simulink model "building_EXAMPLE_v1"  (R2016b)
settings: Solver=ode23tb  StartTime=-building.preruntime+8760*3600  StopTime=building.runtime+8760*3600  MaxStep=600  EnableMultiTasking=on
StartFcn:
  | tic
StopFcn:
  | toc
values from neighbouring files (symbols this model uses):
  building = create_building_automatic(building, modify, import_mode, name_XML, name_EXCEL, name_PHPP, NUMBEROFZONES)    [work_EXAMPLE_v1.m]
undefined symbols (not defined in the file or in its folder): A, B, C, cp, Dd, Dreifach, FluidMix, get_building, ID, MassFlow, p, Pressure, Qdot_C, Qdot_C_energy, Qdot_H, Qdot_H_energy, Qdot_I_electricity, Qdot_I_electricity_energy, Qdot_I_light, Qdot_I_light_energy, Qdot_I_person, Qdot_I_person_energy, Qdot_S, Qdot_S_energy, Qdot_T_ground, Qdot_T_ground_energy, Qdot_T_neighbour, Qdot_T_neighbour_energy, Qdot_T_opaque, Qdot_T_opaque_energy, Qdot_T_window, Qdot_T_window_energy, Qdot_V_infiltration, Qdot_V_infiltration_energy, Qdot_V_mech, Qdot_V_mech_energy, Qdot_V_window, Qdot_V_window_energy, rho, Tc, Temperature, Tr, Ts, Wärmeschutzglas, x_CO2, x_H2O, x_VOC
libraries: carnotUIBK x1931, carnot x83, simulink_extras x22, simulink x12
(part 8 of 35)

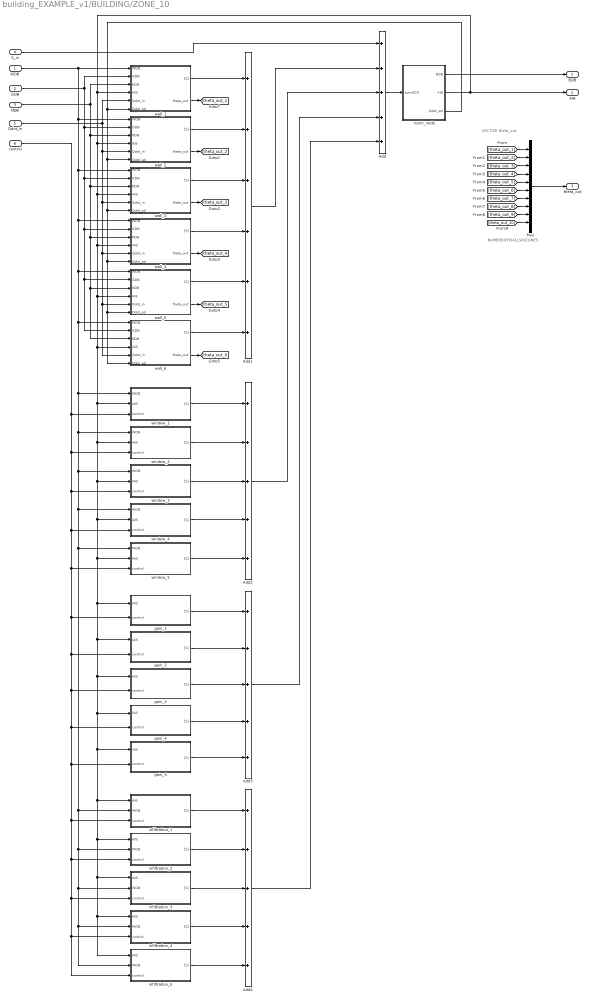
== system building_EXAMPLE_v1/BUILDING/ZONE_10 ==
  note: VECTOR theta_out
  note: NUMBEROFWALLSINZONES
  WDB : Inport
  GDB : Inport  Port=2
  NDB : Inport  Port=3
  S_in : Inport  Port=4
  Qdot_in : Inport  Port=5
  control : Inport  Port=6
  Add{,2..4} (4 alike) : Sum  Inputs=5
  Add1 : Sum  Inputs=6
  Mux : Mux  Inputs=10
  gain_1 : Subsystem  Variant=on  mask{zone=z.matrix_gains, gains=b.gains, subgain=1}
      mask init: same as building_EXAMPLE_v1/BUILDING/ZONE_1/gain_1
      mask Display:
      | fprintf('GAINS:\n')
      | fprintf('\n%s', ga.name)
  gain_2 : Subsystem  Variant=on  mask{zone=z.matrix_gains, gains=b.gains, subgain=2}
      mask init: same as building_EXAMPLE_v1/BUILDING/ZONE_1/gain_1
      mask Display:
      | fprintf('GAINS:\n')
      | fprintf('\n%s', ga.name)
  gain_3 : Subsystem  Variant=on  mask{zone=z.matrix_gains, gains=b.gains, subgain=3}
      mask init: same as building_EXAMPLE_v1/BUILDING/ZONE_1/gain_1
      mask Display:
      | fprintf('GAINS:\n')
      | fprintf('\n%s', ga.name)
  gain_4 : Subsystem  Variant=on  mask{zone=z.matrix_gains, gains=b.gains, subgain=4}
      mask init: same as building_EXAMPLE_v1/BUILDING/ZONE_1/gain_1
      mask Display:
      | fprintf('GAINS:\n')
      | fprintf('\n%s', ga.name)
  gain_5 : Subsystem  Variant=on  mask{zone=z.matrix_gains, gains=b.gains, subgain=4}
      mask init: same as building_EXAMPLE_v1/BUILDING/ZONE_1/gain_1
      mask Display:
      | fprintf('GAINS:\n')
      | fprintf('\n%s', ga.name)
  infiltration_1 : Subsystem  Variant=on  mask{zone=z.matrix_wi, window=1}
      mask init: same as building_EXAMPLE_v1/BUILDING/ZONE_1/infiltration_1
      mask Display:
      | fprintf('INFILTRATION:\n')
      | %fprintf('\n%s', const.name)
  infiltration_2 : Subsystem  Variant=on  mask{zone=z.matrix_wi, window=2}
      mask init: same as building_EXAMPLE_v1/BUILDING/ZONE_1/infiltration_1
      mask Display:
      | fprintf('INFILTRATION:\n')
      | %fprintf('\n%s', const.name)
  infiltration_3 : Subsystem  Variant=on  mask{zone=z.matrix_wi, window=3}
      mask init: same as building_EXAMPLE_v1/BUILDING/ZONE_1/infiltration_1
      mask Display:
      | fprintf('INFILTRATION:\n')
      | %fprintf('\n%s', const.name)
  infiltration_4 : Subsystem  Variant=on  mask{zone=z.matrix_wi, window=4}
      mask init: same as building_EXAMPLE_v1/BUILDING/ZONE_1/infiltration_1
      mask Display:
      | fprintf('INFILTRATION:\n')
      | %fprintf('\n%s', const.name)
  infiltration_5 : Subsystem  Variant=on  mask{zone=z.matrix_wi, window=5}
      mask init: same as building_EXAMPLE_v1/BUILDING/ZONE_1/infiltration_1
      mask Display:
      | fprintf('INFILTRATION:\n')
      | %fprintf('\n%s', const.name)
  room_node : Subsystem  Variant=on
  wall_1 : Subsystem  Variant=on  mask{zone=z.matrix_wd, construction=b.construction, wall=1}
      mask init: same as building_EXAMPLE_v1/BUILDING/ZONE_1/wall_1
      mask Display:
      | fprintf('CONSTRUCTION:\n')
      | fprintf('\n%s', const.name)
  wall_2 : Subsystem  Variant=on  mask{zone=z.matrix_wd, construction=b.construction, wall=2}
      mask init: same as building_EXAMPLE_v1/BUILDING/ZONE_1/wall_1
      mask Display:
      | fprintf('CONSTRUCTION:\n')
      | fprintf('\n%s', const.name)
  wall_3 : Subsystem  Variant=on  mask{zone=z.matrix_wd, construction=b.construction, wall=3}
      mask init: same as building_EXAMPLE_v1/BUILDING/ZONE_1/wall_1
      mask Display:
      | fprintf('CONSTRUCTION:\n')
      | fprintf('\n%s', const.name)
  wall_4 : Subsystem  Variant=on  mask{zone=z.matrix_wd, construction=b.construction, wall=4}
      mask init: same as building_EXAMPLE_v1/BUILDING/ZONE_1/wall_1
      mask Display:
      | fprintf('CONSTRUCTION:\n')
      | fprintf('\n%s', const.name)
  wall_5 : Subsystem  Variant=on  mask{zone=z.matrix_wd, construction=b.construction, wall=5}
      mask init: same as building_EXAMPLE_v1/BUILDING/ZONE_1/wall_1
      mask Display:
      | fprintf('CONSTRUCTION:\n')
      | fprintf('\n%s', const.name)
  wall_6 : Subsystem  Variant=on  mask{zone=z.matrix_wd, construction=b.construction, wall=6}
      mask init: same as building_EXAMPLE_v1/BUILDING/ZONE_1/wall_1
      mask Display:
      | fprintf('CONSTRUCTION:\n')
      | fprintf('\n%s', const.name)
  window_1 : Subsystem  Variant=on  mask{zone=z.matrix_wi, construction=b.construction, window=1}
      mask init: same as building_EXAMPLE_v1/BUILDING/ZONE_1/window_1
      mask Display:
      | fprintf('CONSTRUCTION:\n')
      | fprintf('\n%s', const.name)
  window_2 : Subsystem  Variant=on  mask{zone=z.matrix_wi, construction=b.construction, window=2}
      mask init: same as building_EXAMPLE_v1/BUILDING/ZONE_1/window_1
      mask Display:
      | fprintf('CONSTRUCTION:\n')
      | fprintf('\n%s', const.name)
  window_3 : Subsystem  Variant=on  mask{zone=z.matrix_wi, construction=b.construction, window=3}
      mask init: same as building_EXAMPLE_v1/BUILDING/ZONE_1/window_1
      mask Display:
      | fprintf('CONSTRUCTION:\n')
      | fprintf('\n%s', const.name)
  window_4 : Subsystem  Variant=on  mask{zone=z.matrix_wi, construction=b.construction, window=4}
      mask init: same as building_EXAMPLE_v1/BUILDING/ZONE_1/window_1
      mask Display:
      | fprintf('CONSTRUCTION:\n')
      | fprintf('\n%s', const.name)
  window_5 : Subsystem  Variant=on  mask{zone=z.matrix_wi, construction=b.construction, window=5}
      mask init: same as building_EXAMPLE_v1/BUILDING/ZONE_1/window_1
      mask Display:
      | fprintf('CONSTRUCTION:\n')
      | fprintf('\n%s', const.name)
  BDB : Outport
  AIB : Outport  Port=2
  theta_out : Outport  Port=3
  wires:
  WDB/1 -> wall_3/1(WDB), wall_4/1(WDB), wall_5/1(WDB), wall_6/1(WDB), window_1/1(WDB), window_4/1(WDB), infiltration_2/2(WDB), infiltration_3/2(WDB), infiltration_4/2(WDB), infiltration_5/2(WDB), infiltration_1/2(WDB), window_5/1(WDB), window_3/1(WDB), window_2/1(WDB), wall_2/1(WDB), wall_1/1(WDB)
  room_node/1(BDB) -> BDB/1
  S_in/1 -> Add/1
  Qdot_in/1 -> wall_1/5(Qdot_in), wall_3/5(Qdot_in), wall_4/5(Qdot_in), wall_6/5(Qdot_in), wall_5/5(Qdot_in), wall_2/5(Qdot_in)
  Add/1 -> room_node/1(sum([S]))
  room_node/3(Qdot_sol) -> wall_3/6(Qdot_sol), wall_4/6(Qdot_sol), wall_6/6(Qdot_sol), wall_5/6(Qdot_sol), wall_2/6(Qdot_sol), wall_1/6(Qdot_sol)
  wall_1/2(theta_out) -> [theta_out_1]
  control/1 -> gain_2/2(control), gain_3/2(control), infiltration_1/3(control), infiltration_2/3(control), infiltration_3/3(control), infiltration_4/3(control), infiltration_5/3(control), gain_5/2(control), gain_4/2(control), gain_1/2(control), window_5/3(control), window_4/3(control), window_3/3(control), window_2/3(control), window_1/3(control)
  room_node/2(AIB) -> AIB/1, wall_3/4(AIB), wall_4/4(AIB), wall_5/4(AIB), wall_6/4(AIB), gain_2/1(AIB), gain_3/1(AIB), infiltration_2/1(AIB), infiltration_3/1(AIB), infiltration_4/1(AIB), infiltration_5/1(AIB), infiltration_1/1(AIB), gain_5/1(AIB), gain_4/1(AIB), gain_1/1(AIB), window_5/2(AIB), window_4/2(AIB), window_3/2(AIB), window_2/2(AIB), window_1/2(AIB), wall_2/4(AIB), wall_1/4(AIB)
  Mux/1 -> theta_out/1
  [theta_out_1] -> Mux/1
  [theta_out_2] -> Mux/2
  [theta_out_10] -> Mux/10
  [theta_out_9] -> Mux/9
  [theta_out_8] -> Mux/8
  [theta_out_7] -> Mux/7
  [theta_out_6] -> Mux/6
  [theta_out_5] -> Mux/5
  [theta_out_4] -> Mux/4
  [theta_out_3] -> Mux/3
  wall_2/2(theta_out) -> [theta_out_2]
  GDB/1 -> wall_1/2(GDB), wall_3/2(GDB), wall_4/2(GDB), wall_6/2(GDB), wall_5/2(GDB), wall_2/2(GDB)
  wall_3/2(theta_out) -> [theta_out_3]
  wall_4/2(theta_out) -> [theta_out_4]
  wall_5/2(theta_out) -> [theta_out_5]
  wall_6/2(theta_out) -> [theta_out_6]
  NDB/1 -> wall_1/3(NDB), wall_3/3(NDB), wall_4/3(NDB), wall_6/3(NDB), wall_5/3(NDB), wall_2/3(NDB)
  wall_1/1("[S]") -> Add1/1
  wall_6/1("[S]") -> Add1/6
  wall_2/1("[S]") -> Add1/2
  wall_3/1("[S]") -> Add1/3
  wall_4/1("[S]") -> Add1/4
  wall_5/1("[S]") -> Add1/5
  Add1/1 -> Add/2
  window_1/1("[S]") -> Add2/1
  window_5/1("[S]") -> Add2/5
  window_2/1("[S]") -> Add2/2
  window_3/1("[S]") -> Add2/3
  window_4/1("[S]") -> Add2/4
  Add2/1 -> Add/3
  gain_1/1("[S]") -> Add3/1
  gain_5/1("[S]") -> Add3/5
  gain_2/1("[S]") -> Add3/2
  gain_3/1("[S]") -> Add3/3
  gain_4/1("[S]") -> Add3/4
  Add3/1 -> Add/4
  infiltration_1/1("[S]") -> Add4/1
  infiltration_5/1("[S]") -> Add4/5
  infiltration_4/1("[S]") -> Add4/4
  infiltration_3/1("[S]") -> Add4/3
  infiltration_2/1("[S]") -> Add4/2
  Add4/1 -> Add/5

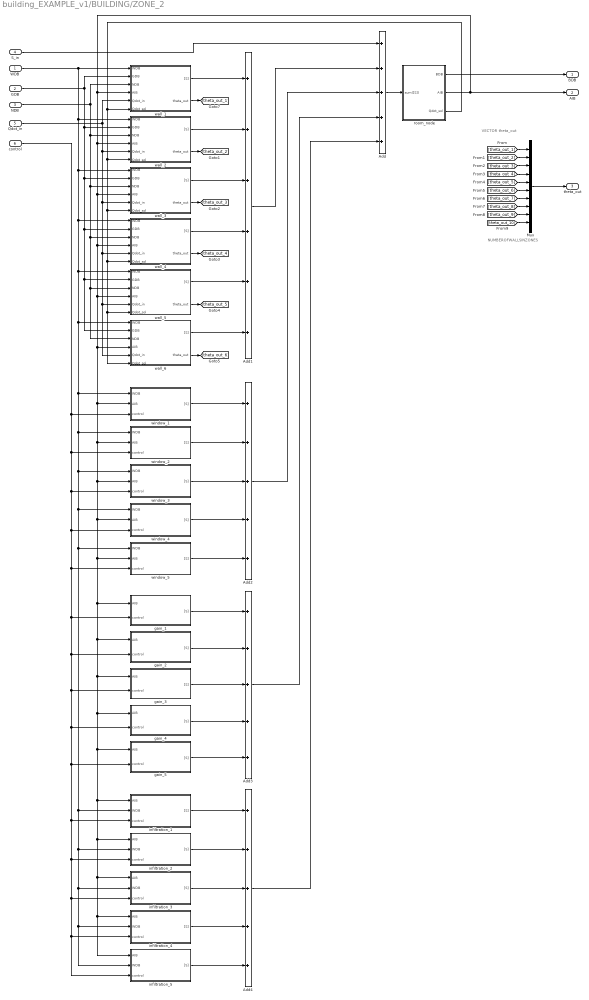
== system building_EXAMPLE_v1/BUILDING/ZONE_2 ==
  note: VECTOR theta_out
  note: NUMBEROFWALLSINZONES
  WDB : Inport
  GDB : Inport  Port=2
  NDB : Inport  Port=3
  S_in : Inport  Port=4
  Qdot_in : Inport  Port=5
  control : Inport  Port=6
  Add{,2..4} (4 alike) : Sum  Inputs=5
  Add1 : Sum  Inputs=6
  Mux : Mux  Inputs=10
  gain_1 : Subsystem  Variant=on  mask{zone=z.matrix_gains, gains=b.gains, subgain=1}
      mask init: same as building_EXAMPLE_v1/BUILDING/ZONE_1/gain_1
      mask Display:
      | fprintf('GAINS:\n')
      | fprintf('\n%s', ga.name)
  gain_2 : Subsystem  Variant=on  mask{zone=z.matrix_gains, gains=b.gains, subgain=2}
      mask init: same as building_EXAMPLE_v1/BUILDING/ZONE_1/gain_1
      mask Display:
      | fprintf('GAINS:\n')
      | fprintf('\n%s', ga.name)
  gain_3 : Subsystem  Variant=on  mask{zone=z.matrix_gains, gains=b.gains, subgain=3}
      mask init: same as building_EXAMPLE_v1/BUILDING/ZONE_1/gain_1
      mask Display:
      | fprintf('GAINS:\n')
      | fprintf('\n%s', ga.name)
  gain_4 : Subsystem  Variant=on  mask{zone=z.matrix_gains, gains=b.gains, subgain=4}
      mask init: same as building_EXAMPLE_v1/BUILDING/ZONE_1/gain_1
      mask Display:
      | fprintf('GAINS:\n')
      | fprintf('\n%s', ga.name)
  gain_5 : Subsystem  Variant=on  mask{zone=z.matrix_gains, gains=b.gains, subgain=4}
      mask init: same as building_EXAMPLE_v1/BUILDING/ZONE_1/gain_1
      mask Display:
      | fprintf('GAINS:\n')
      | fprintf('\n%s', ga.name)
  infiltration_1 : Subsystem  Variant=on  mask{zone=z.matrix_wi, window=1}
      mask init: same as building_EXAMPLE_v1/BUILDING/ZONE_1/infiltration_1
      mask Display:
      | fprintf('INFILTRATION:\n')
      | %fprintf('\n%s', const.name)
  infiltration_2 : Subsystem  Variant=on  mask{zone=z.matrix_wi, window=2}
      mask init: same as building_EXAMPLE_v1/BUILDING/ZONE_1/infiltration_1
      mask Display:
      | fprintf('INFILTRATION:\n')
      | %fprintf('\n%s', const.name)
  infiltration_3 : Subsystem  Variant=on  mask{zone=z.matrix_wi, window=3}
      mask init: same as building_EXAMPLE_v1/BUILDING/ZONE_1/infiltration_1
      mask Display:
      | fprintf('INFILTRATION:\n')
      | %fprintf('\n%s', const.name)
  infiltration_4 : Subsystem  Variant=on  mask{zone=z.matrix_wi, window=4}
      mask init: same as building_EXAMPLE_v1/BUILDING/ZONE_1/infiltration_1
      mask Display:
      | fprintf('INFILTRATION:\n')
      | %fprintf('\n%s', const.name)
  infiltration_5 : Subsystem  Variant=on  mask{zone=z.matrix_wi, window=5}
      mask init: same as building_EXAMPLE_v1/BUILDING/ZONE_1/infiltration_1
      mask Display:
      | fprintf('INFILTRATION:\n')
      | %fprintf('\n%s', const.name)
  room_node : Subsystem  Variant=on
  wall_1 : Subsystem  Variant=on  mask{zone=z.matrix_wd, construction=b.construction, wall=1}
      mask init: same as building_EXAMPLE_v1/BUILDING/ZONE_1/wall_1
      mask Display:
      | fprintf('CONSTRUCTION:\n')
      | fprintf('\n%s', const.name)
  wall_2 : Subsystem  Variant=on  mask{zone=z.matrix_wd, construction=b.construction, wall=2}
      mask init: same as building_EXAMPLE_v1/BUILDING/ZONE_1/wall_1
      mask Display:
      | fprintf('CONSTRUCTION:\n')
      | fprintf('\n%s', const.name)
  wall_3 : Subsystem  Variant=on  mask{zone=z.matrix_wd, construction=b.construction, wall=3}
      mask init: same as building_EXAMPLE_v1/BUILDING/ZONE_1/wall_1
      mask Display:
      | fprintf('CONSTRUCTION:\n')
      | fprintf('\n%s', const.name)
  wall_4 : Subsystem  Variant=on  mask{zone=z.matrix_wd, construction=b.construction, wall=4}
      mask init: same as building_EXAMPLE_v1/BUILDING/ZONE_1/wall_1
      mask Display:
      | fprintf('CONSTRUCTION:\n')
      | fprintf('\n%s', const.name)
  wall_5 : Subsystem  Variant=on  mask{zone=z.matrix_wd, construction=b.construction, wall=5}
      mask init: same as building_EXAMPLE_v1/BUILDING/ZONE_1/wall_1
      mask Display:
      | fprintf('CONSTRUCTION:\n')
      | fprintf('\n%s', const.name)
  wall_6 : Subsystem  Variant=on  mask{zone=z.matrix_wd, construction=b.construction, wall=6}
      mask init: same as building_EXAMPLE_v1/BUILDING/ZONE_1/wall_1
      mask Display:
      | fprintf('CONSTRUCTION:\n')
      | fprintf('\n%s', const.name)
  window_1 : Subsystem  Variant=on  mask{zone=z.matrix_wi, construction=b.construction, window=1}
      mask init: same as building_EXAMPLE_v1/BUILDING/ZONE_1/window_1
      mask Display:
      | fprintf('CONSTRUCTION:\n')
      | fprintf('\n%s', const.name)
  window_2 : Subsystem  Variant=on  mask{zone=z.matrix_wi, construction=b.construction, window=2}
      mask init: same as building_EXAMPLE_v1/BUILDING/ZONE_1/window_1
      mask Display:
      | fprintf('CONSTRUCTION:\n')
      | fprintf('\n%s', const.name)
  window_3 : Subsystem  Variant=on  mask{zone=z.matrix_wi, construction=b.construction, window=3}
      mask init: same as building_EXAMPLE_v1/BUILDING/ZONE_1/window_1
      mask Display:
      | fprintf('CONSTRUCTION:\n')
      | fprintf('\n%s', const.name)
  window_4 : Subsystem  Variant=on  mask{zone=z.matrix_wi, construction=b.construction, window=4}
      mask init: same as building_EXAMPLE_v1/BUILDING/ZONE_1/window_1
      mask Display:
      | fprintf('CONSTRUCTION:\n')
      | fprintf('\n%s', const.name)
  window_5 : Subsystem  Variant=on  mask{zone=z.matrix_wi, construction=b.construction, window=5}
      mask init: same as building_EXAMPLE_v1/BUILDING/ZONE_1/window_1
      mask Display:
      | fprintf('CONSTRUCTION:\n')
      | fprintf('\n%s', const.name)
  BDB : Outport
  AIB : Outport  Port=2
  theta_out : Outport  Port=3
  wires:
  WDB/1 -> wall_3/1(WDB), wall_4/1(WDB), wall_5/1(WDB), wall_6/1(WDB), window_1/1(WDB), window_4/1(WDB), infiltration_2/2(WDB), infiltration_3/2(WDB), infiltration_4/2(WDB), infiltration_5/2(WDB), infiltration_1/2(WDB), window_5/1(WDB), window_3/1(WDB), window_2/1(WDB), wall_2/1(WDB), wall_1/1(WDB)
  room_node/1(BDB) -> BDB/1
  S_in/1 -> Add/1
  Qdot_in/1 -> wall_1/5(Qdot_in), wall_3/5(Qdot_in), wall_4/5(Qdot_in), wall_6/5(Qdot_in), wall_5/5(Qdot_in), wall_2/5(Qdot_in)
  Add/1 -> room_node/1(sum([S]))
  room_node/3(Qdot_sol) -> wall_3/6(Qdot_sol), wall_4/6(Qdot_sol), wall_6/6(Qdot_sol), wall_5/6(Qdot_sol), wall_2/6(Qdot_sol), wall_1/6(Qdot_sol)
  wall_1/2(theta_out) -> [theta_out_1]
  control/1 -> gain_2/2(control), gain_3/2(control), infiltration_1/3(control), infiltration_2/3(control), infiltration_3/3(control), infiltration_4/3(control), infiltration_5/3(control), gain_5/2(control), gain_4/2(control), gain_1/2(control), window_5/3(control), window_4/3(control), window_3/3(control), window_2/3(control), window_1/3(control)
  room_node/2(AIB) -> AIB/1, wall_3/4(AIB), wall_4/4(AIB), wall_5/4(AIB), wall_6/4(AIB), gain_2/1(AIB), gain_3/1(AIB), infiltration_2/1(AIB), infiltration_3/1(AIB), infiltration_4/1(AIB), infiltration_5/1(AIB), infiltration_1/1(AIB), gain_5/1(AIB), gain_4/1(AIB), gain_1/1(AIB), window_5/2(AIB), window_4/2(AIB), window_3/2(AIB), window_2/2(AIB), window_1/2(AIB), wall_2/4(AIB), wall_1/4(AIB)
  Mux/1 -> theta_out/1
  [theta_out_1] -> Mux/1
  [theta_out_2] -> Mux/2
  [theta_out_10] -> Mux/10
  [theta_out_9] -> Mux/9
  [theta_out_8] -> Mux/8
  [theta_out_7] -> Mux/7
  [theta_out_6] -> Mux/6
  [theta_out_5] -> Mux/5
  [theta_out_4] -> Mux/4
  [theta_out_3] -> Mux/3
  wall_2/2(theta_out) -> [theta_out_2]
  GDB/1 -> wall_1/2(GDB), wall_3/2(GDB), wall_4/2(GDB), wall_6/2(GDB), wall_5/2(GDB), wall_2/2(GDB)
  wall_3/2(theta_out) -> [theta_out_3]
  wall_4/2(theta_out) -> [theta_out_4]
  wall_5/2(theta_out) -> [theta_out_5]
  wall_6/2(theta_out) -> [theta_out_6]
  NDB/1 -> wall_1/3(NDB), wall_3/3(NDB), wall_4/3(NDB), wall_6/3(NDB), wall_5/3(NDB), wall_2/3(NDB)
  wall_1/1("[S]") -> Add1/1
  wall_6/1("[S]") -> Add1/6
  wall_2/1("[S]") -> Add1/2
  wall_3/1("[S]") -> Add1/3
  wall_4/1("[S]") -> Add1/4
  wall_5/1("[S]") -> Add1/5
  Add1/1 -> Add/2
  window_1/1("[S]") -> Add2/1
  window_5/1("[S]") -> Add2/5
  window_2/1("[S]") -> Add2/2
  window_3/1("[S]") -> Add2/3
  window_4/1("[S]") -> Add2/4
  Add2/1 -> Add/3
  gain_1/1("[S]") -> Add3/1
  gain_5/1("[S]") -> Add3/5
  gain_2/1("[S]") -> Add3/2
  gain_3/1("[S]") -> Add3/3
  gain_4/1("[S]") -> Add3/4
  Add3/1 -> Add/4
  infiltration_1/1("[S]") -> Add4/1
  infiltration_5/1("[S]") -> Add4/5
  infiltration_4/1("[S]") -> Add4/4
  infiltration_3/1("[S]") -> Add4/3
  infiltration_2/1("[S]") -> Add4/2
  Add4/1 -> Add/5

== system building_EXAMPLE_v1/BUILDING/ZONE_3 ==
  note: VECTOR theta_out
  note: NUMBEROFWALLSINZONES
  WDB : Inport
  GDB : Inport  Port=2
  NDB : Inport  Port=3
  S_in : Inport  Port=4
  Qdot_in : Inport  Port=5
  control : Inport  Port=6
  Add{,2..4} (4 alike) : Sum  Inputs=5
  Add1 : Sum  Inputs=6
  Mux : Mux  Inputs=10
  gain_1 : Subsystem  Variant=on  mask{zone=z.matrix_gains, gains=b.gains, subgain=1}
      mask init: same as building_EXAMPLE_v1/BUILDING/ZONE_1/gain_1
      mask Display:
      | fprintf('GAINS:\n')
      | fprintf('\n%s', ga.name)
  gain_2 : Subsystem  Variant=on  mask{zone=z.matrix_gains, gains=b.gains, subgain=2}
      mask init: same as building_EXAMPLE_v1/BUILDING/ZONE_1/gain_1
      mask Display:
      | fprintf('GAINS:\n')
      | fprintf('\n%s', ga.name)
  gain_3 : Subsystem  Variant=on  mask{zone=z.matrix_gains, gains=b.gains, subgain=3}
      mask init: same as building_EXAMPLE_v1/BUILDING/ZONE_1/gain_1
      mask Display:
      | fprintf('GAINS:\n')
      | fprintf('\n%s', ga.name)
  gain_4 : Subsystem  Variant=on  mask{zone=z.matrix_gains, gains=b.gains, subgain=4}
      mask init: same as building_EXAMPLE_v1/BUILDING/ZONE_1/gain_1
      mask Display:
      | fprintf('GAINS:\n')
      | fprintf('\n%s', ga.name)
  gain_5 : Subsystem  Variant=on  mask{zone=z.matrix_gains, gains=b.gains, subgain=4}
      mask init: same as building_EXAMPLE_v1/BUILDING/ZONE_1/gain_1
      mask Display:
      | fprintf('GAINS:\n')
      | fprintf('\n%s', ga.name)
  infiltration_1 : Subsystem  Variant=on  mask{zone=z.matrix_wi, window=1}
      mask init: same as building_EXAMPLE_v1/BUILDING/ZONE_1/infiltration_1
      mask Display:
      | fprintf('INFILTRATION:\n')
      | %fprintf('\n%s', const.name)
  infiltration_2 : Subsystem  Variant=on  mask{zone=z.matrix_wi, window=2}
      mask init: same as building_EXAMPLE_v1/BUILDING/ZONE_1/infiltration_1
      mask Display:
      | fprintf('INFILTRATION:\n')
      | %fprintf('\n%s', const.name)
  infiltration_3 : Subsystem  Variant=on  mask{zone=z.matrix_wi, window=3}
      mask init: same as building_EXAMPLE_v1/BUILDING/ZONE_1/infiltration_1
      mask Display:
      | fprintf('INFILTRATION:\n')
      | %fprintf('\n%s', const.name)
  infiltration_4 : Subsystem  Variant=on  mask{zone=z.matrix_wi, window=4}
      mask init: same as building_EXAMPLE_v1/BUILDING/ZONE_1/infiltration_1
      mask Display:
      | fprintf('INFILTRATION:\n')
      | %fprintf('\n%s', const.name)
  infiltration_5 : Subsystem  Variant=on  mask{zone=z.matrix_wi, window=5}
      mask init: same as building_EXAMPLE_v1/BUILDING/ZONE_1/infiltration_1
      mask Display:
      | fprintf('INFILTRATION:\n')
      | %fprintf('\n%s', const.name)
  room_node : Subsystem  Variant=on
  wall_1 : Subsystem  Variant=on  mask{zone=z.matrix_wd, construction=b.construction, wall=1}
      mask init: same as building_EXAMPLE_v1/BUILDING/ZONE_1/wall_1
      mask Display:
      | fprintf('CONSTRUCTION:\n')
      | fprintf('\n%s', const.name)
  wall_2 : Subsystem  Variant=on  mask{zone=z.matrix_wd, construction=b.construction, wall=2}
      mask init: same as building_EXAMPLE_v1/BUILDING/ZONE_1/wall_1
      mask Display:
      | fprintf('CONSTRUCTION:\n')
      | fprintf('\n%s', const.name)
  wall_3 : Subsystem  Variant=on  mask{zone=z.matrix_wd, construction=b.construction, wall=3}
      mask init: same as building_EXAMPLE_v1/BUILDING/ZONE_1/wall_1
      mask Display:
      | fprintf('CONSTRUCTION:\n')
      | fprintf('\n%s', const.name)
  wall_4 : Subsystem  Variant=on  mask{zone=z.matrix_wd, construction=b.construction, wall=4}
      mask init: same as building_EXAMPLE_v1/BUILDING/ZONE_1/wall_1
      mask Display:
      | fprintf('CONSTRUCTION:\n')
      | fprintf('\n%s', const.name)
  wall_5 : Subsystem  Variant=on  mask{zone=z.matrix_wd, construction=b.construction, wall=5}
      mask init: same as building_EXAMPLE_v1/BUILDING/ZONE_1/wall_1
      mask Display:
      | fprintf('CONSTRUCTION:\n')
      | fprintf('\n%s', const.name)
  wall_6 : Subsystem  Variant=on  mask{zone=z.matrix_wd, construction=b.construction, wall=6}
      mask init: same as building_EXAMPLE_v1/BUILDING/ZONE_1/wall_1
      mask Display:
      | fprintf('CONSTRUCTION:\n')
      | fprintf('\n%s', const.name)
  window_1 : Subsystem  Variant=on  mask{zone=z.matrix_wi, construction=b.construction, window=1}
      mask init: same as building_EXAMPLE_v1/BUILDING/ZONE_1/window_1
      mask Display:
      | fprintf('CONSTRUCTION:\n')
      | fprintf('\n%s', const.name)
  window_2 : Subsystem  Variant=on  mask{zone=z.matrix_wi, construction=b.construction, window=2}
      mask init: same as building_EXAMPLE_v1/BUILDING/ZONE_1/window_1
      mask Display:
      | fprintf('CONSTRUCTION:\n')
      | fprintf('\n%s', const.name)
  window_3 : Subsystem  Variant=on  mask{zone=z.matrix_wi, construction=b.construction, window=3}
      mask init: same as building_EXAMPLE_v1/BUILDING/ZONE_1/window_1
      mask Display:
      | fprintf('CONSTRUCTION:\n')
      | fprintf('\n%s', const.name)
  window_4 : Subsystem  Variant=on  mask{zone=z.matrix_wi, construction=b.construction, window=4}
      mask init: same as building_EXAMPLE_v1/BUILDING/ZONE_1/window_1
      mask Display:
      | fprintf('CONSTRUCTION:\n')
      | fprintf('\n%s', const.name)
  window_5 : Subsystem  Variant=on  mask{zone=z.matrix_wi, construction=b.construction, window=5}
      mask init: same as building_EXAMPLE_v1/BUILDING/ZONE_1/window_1
      mask Display:
      | fprintf('CONSTRUCTION:\n')
      | fprintf('\n%s', const.name)
  BDB : Outport
  AIB : Outport  Port=2
  theta_out : Outport  Port=3
  wires:
  WDB/1 -> wall_3/1(WDB), wall_4/1(WDB), wall_5/1(WDB), wall_6/1(WDB), window_1/1(WDB), window_4/1(WDB), infiltration_2/2(WDB), infiltration_3/2(WDB), infiltration_4/2(WDB), infiltration_5/2(WDB), infiltration_1/2(WDB), window_5/1(WDB), window_3/1(WDB), window_2/1(WDB), wall_2/1(WDB), wall_1/1(WDB)
  room_node/1(BDB) -> BDB/1
  S_in/1 -> Add/1
  Qdot_in/1 -> wall_1/5(Qdot_in), wall_3/5(Qdot_in), wall_4/5(Qdot_in), wall_6/5(Qdot_in), wall_5/5(Qdot_in), wall_2/5(Qdot_in)
  Add/1 -> room_node/1(sum([S]))
  room_node/3(Qdot_sol) -> wall_3/6(Qdot_sol), wall_4/6(Qdot_sol), wall_6/6(Qdot_sol), wall_5/6(Qdot_sol), wall_2/6(Qdot_sol), wall_1/6(Qdot_sol)
  wall_1/2(theta_out) -> [theta_out_1]
  control/1 -> gain_2/2(control), gain_3/2(control), infiltration_1/3(control), infiltration_2/3(control), infiltration_3/3(control), infiltration_4/3(control), infiltration_5/3(control), gain_5/2(control), gain_4/2(control), gain_1/2(control), window_5/3(control), window_4/3(control), window_3/3(control), window_2/3(control), window_1/3(control)
  room_node/2(AIB) -> AIB/1, wall_3/4(AIB), wall_4/4(AIB), wall_5/4(AIB), wall_6/4(AIB), gain_2/1(AIB), gain_3/1(AIB), infiltration_2/1(AIB), infiltration_3/1(AIB), infiltration_4/1(AIB), infiltration_5/1(AIB), infiltration_1/1(AIB), gain_5/1(AIB), gain_4/1(AIB), gain_1/1(AIB), window_5/2(AIB), window_4/2(AIB), window_3/2(AIB), window_2/2(AIB), window_1/2(AIB), wall_2/4(AIB), wall_1/4(AIB)
  Mux/1 -> theta_out/1
  [theta_out_1] -> Mux/1
  [theta_out_2] -> Mux/2
  [theta_out_10] -> Mux/10
  [theta_out_9] -> Mux/9
  [theta_out_8] -> Mux/8
  [theta_out_7] -> Mux/7
  [theta_out_6] -> Mux/6
  [theta_out_5] -> Mux/5
  [theta_out_4] -> Mux/4
  [theta_out_3] -> Mux/3
  wall_2/2(theta_out) -> [theta_out_2]
  GDB/1 -> wall_1/2(GDB), wall_3/2(GDB), wall_4/2(GDB), wall_6/2(GDB), wall_5/2(GDB), wall_2/2(GDB)
  wall_3/2(theta_out) -> [theta_out_3]
  wall_4/2(theta_out) -> [theta_out_4]
  wall_5/2(theta_out) -> [theta_out_5]
  wall_6/2(theta_out) -> [theta_out_6]
  NDB/1 -> wall_1/3(NDB), wall_3/3(NDB), wall_4/3(NDB), wall_6/3(NDB), wall_5/3(NDB), wall_2/3(NDB)
  wall_1/1("[S]") -> Add1/1
  wall_6/1("[S]") -> Add1/6
  wall_2/1("[S]") -> Add1/2
  wall_3/1("[S]") -> Add1/3
  wall_4/1("[S]") -> Add1/4
  wall_5/1("[S]") -> Add1/5
  Add1/1 -> Add/2
  window_1/1("[S]") -> Add2/1
  window_5/1("[S]") -> Add2/5
  window_2/1("[S]") -> Add2/2
  window_3/1("[S]") -> Add2/3
  window_4/1("[S]") -> Add2/4
  Add2/1 -> Add/3
  gain_1/1("[S]") -> Add3/1
  gain_5/1("[S]") -> Add3/5
  gain_2/1("[S]") -> Add3/2
  gain_3/1("[S]") -> Add3/3
  gain_4/1("[S]") -> Add3/4
  Add3/1 -> Add/4
  infiltration_1/1("[S]") -> Add4/1
  infiltration_5/1("[S]") -> Add4/5
  infiltration_4/1("[S]") -> Add4/4
  infiltration_3/1("[S]") -> Add4/3
  infiltration_2/1("[S]") -> Add4/2
  Add4/1 -> Add/5

== system building_EXAMPLE_v1/BUILDING/ZONE_4 ==
  note: VECTOR theta_out
  note: NUMBEROFWALLSINZONES
  WDB : Inport
  GDB : Inport  Port=2
  NDB : Inport  Port=3
  S_in : Inport  Port=4
  Qdot_in : Inport  Port=5
  control : Inport  Port=6
  Add{,2..4} (4 alike) : Sum  Inputs=5
  Add1 : Sum  Inputs=6
  Mux : Mux  Inputs=10
  gain_1 : Subsystem  Variant=on  mask{zone=z.matrix_gains, gains=b.gains, subgain=1}
      mask init: same as building_EXAMPLE_v1/BUILDING/ZONE_1/gain_1
      mask Display:
      | fprintf('GAINS:\n')
      | fprintf('\n%s', ga.name)
  gain_2 : Subsystem  Variant=on  mask{zone=z.matrix_gains, gains=b.gains, subgain=2}
      mask init: same as building_EXAMPLE_v1/BUILDING/ZONE_1/gain_1
      mask Display:
      | fprintf('GAINS:\n')
      | fprintf('\n%s', ga.name)
  gain_3 : Subsystem  Variant=on  mask{zone=z.matrix_gains, gains=b.gains, subgain=3}
      mask init: same as building_EXAMPLE_v1/BUILDING/ZONE_1/gain_1
      mask Display:
      | fprintf('GAINS:\n')
      | fprintf('\n%s', ga.name)
  gain_4 : Subsystem  Variant=on  mask{zone=z.matrix_gains, gains=b.gains, subgain=4}
      mask init: same as building_EXAMPLE_v1/BUILDING/ZONE_1/gain_1
      mask Display:
      | fprintf('GAINS:\n')
      | fprintf('\n%s', ga.name)
  gain_5 : Subsystem  Variant=on  mask{zone=z.matrix_gains, gains=b.gains, subgain=4}
      mask init: same as building_EXAMPLE_v1/BUILDING/ZONE_1/gain_1
      mask Display:
      | fprintf('GAINS:\n')
      | fprintf('\n%s', ga.name)
  infiltration_1 : Subsystem  Variant=on  mask{zone=z.matrix_wi, window=1}
      mask init: same as building_EXAMPLE_v1/BUILDING/ZONE_1/infiltration_1
      mask Display:
      | fprintf('INFILTRATION:\n')
      | %fprintf('\n%s', const.name)
  infiltration_2 : Subsystem  Variant=on  mask{zone=z.matrix_wi, window=2}
      mask init: same as building_EXAMPLE_v1/BUILDING/ZONE_1/infiltration_1
      mask Display:
      | fprintf('INFILTRATION:\n')
      | %fprintf('\n%s', const.name)
  infiltration_3 : Subsystem  Variant=on  mask{zone=z.matrix_wi, window=3}
      mask init: same as building_EXAMPLE_v1/BUILDING/ZONE_1/infiltration_1
      mask Display:
      | fprintf('INFILTRATION:\n')
      | %fprintf('\n%s', const.name)
  infiltration_4 : Subsystem  Variant=on  mask{zone=z.matrix_wi, window=4}
      mask init: same as building_EXAMPLE_v1/BUILDING/ZONE_1/infiltration_1
      mask Display:
      | fprintf('INFILTRATION:\n')
      | %fprintf('\n%s', const.name)
  infiltration_5 : Subsystem  Variant=on  mask{zone=z.matrix_wi, window=5}
      mask init: same as building_EXAMPLE_v1/BUILDING/ZONE_1/infiltration_1
      mask Display:
      | fprintf('INFILTRATION:\n')
      | %fprintf('\n%s', const.name)
  room_node : Subsystem  Variant=on
  wall_1 : Subsystem  Variant=on  mask{zone=z.matrix_wd, construction=b.construction, wall=1}
      mask init: same as building_EXAMPLE_v1/BUILDING/ZONE_1/wall_1
      mask Display:
      | fprintf('CONSTRUCTION:\n')
      | fprintf('\n%s', const.name)
  wall_2 : Subsystem  Variant=on  mask{zone=z.matrix_wd, construction=b.construction, wall=2}
      mask init: same as building_EXAMPLE_v1/BUILDING/ZONE_1/wall_1
      mask Display:
      | fprintf('CONSTRUCTION:\n')
      | fprintf('\n%s', const.name)
  wall_3 : Subsystem  Variant=on  mask{zone=z.matrix_wd, construction=b.construction, wall=3}
      mask init: same as building_EXAMPLE_v1/BUILDING/ZONE_1/wall_1
      mask Display:
      | fprintf('CONSTRUCTION:\n')
      | fprintf('\n%s', const.name)
  wall_4 : Subsystem  Variant=on  mask{zone=z.matrix_wd, construction=b.construction, wall=4}
      mask init: same as building_EXAMPLE_v1/BUILDING/ZONE_1/wall_1
      mask Display:
      | fprintf('CONSTRUCTION:\n')
      | fprintf('\n%s', const.name)
  wall_5 : Subsystem  Variant=on  mask{zone=z.matrix_wd, construction=b.construction, wall=5}
      mask init: same as building_EXAMPLE_v1/BUILDING/ZONE_1/wall_1
      mask Display:
      | fprintf('CONSTRUCTION:\n')
      | fprintf('\n%s', const.name)
  wall_6 : Subsystem  Variant=on  mask{zone=z.matrix_wd, construction=b.construction, wall=6}
      mask init: same as building_EXAMPLE_v1/BUILDING/ZONE_1/wall_1
      mask Display:
      | fprintf('CONSTRUCTION:\n')
      | fprintf('\n%s', const.name)
  window_1 : Subsystem  Variant=on  mask{zone=z.matrix_wi, construction=b.construction, window=1}
      mask init: same as building_EXAMPLE_v1/BUILDING/ZONE_1/window_1
      mask Display:
      | fprintf('CONSTRUCTION:\n')
      | fprintf('\n%s', const.name)
  window_2 : Subsystem  Variant=on  mask{zone=z.matrix_wi, construction=b.construction, window=2}
      mask init: same as building_EXAMPLE_v1/BUILDING/ZONE_1/window_1
      mask Display:
      | fprintf('CONSTRUCTION:\n')
      | fprintf('\n%s', const.name)
  window_3 : Subsystem  Variant=on  mask{zone=z.matrix_wi, construction=b.construction, window=3}
      mask init: same as building_EXAMPLE_v1/BUILDING/ZONE_1/window_1
      mask Display:
      | fprintf('CONSTRUCTION:\n')
      | fprintf('\n%s', const.name)
  window_4 : Subsystem  Variant=on  mask{zone=z.matrix_wi, construction=b.construction, window=4}
      mask init: same as building_EXAMPLE_v1/BUILDING/ZONE_1/window_1
      mask Display:
      | fprintf('CONSTRUCTION:\n')
      | fprintf('\n%s', const.name)
  window_5 : Subsystem  Variant=on  mask{zone=z.matrix_wi, construction=b.construction, window=5}
      mask init: same as building_EXAMPLE_v1/BUILDING/ZONE_1/window_1
      mask Display:
      | fprintf('CONSTRUCTION:\n')
      | fprintf('\n%s', const.name)
  BDB : Outport
  AIB : Outport  Port=2
  theta_out : Outport  Port=3
  wires:
  WDB/1 -> wall_3/1(WDB), wall_4/1(WDB), wall_5/1(WDB), wall_6/1(WDB), window_1/1(WDB), window_4/1(WDB), infiltration_2/2(WDB), infiltration_3/2(WDB), infiltration_4/2(WDB), infiltration_5/2(WDB), infiltration_1/2(WDB), window_5/1(WDB), window_3/1(WDB), window_2/1(WDB), wall_2/1(WDB), wall_1/1(WDB)
  room_node/1(BDB) -> BDB/1
  S_in/1 -> Add/1
  Qdot_in/1 -> wall_1/5(Qdot_in), wall_3/5(Qdot_in), wall_4/5(Qdot_in), wall_6/5(Qdot_in), wall_5/5(Qdot_in), wall_2/5(Qdot_in)
  Add/1 -> room_node/1(sum([S]))
  room_node/3(Qdot_sol) -> wall_3/6(Qdot_sol), wall_4/6(Qdot_sol), wall_6/6(Qdot_sol), wall_5/6(Qdot_sol), wall_2/6(Qdot_sol), wall_1/6(Qdot_sol)
  wall_1/2(theta_out) -> [theta_out_1]
  control/1 -> gain_2/2(control), gain_3/2(control), infiltration_1/3(control), infiltration_2/3(control), infiltration_3/3(control), infiltration_4/3(control), infiltration_5/3(control), gain_5/2(control), gain_4/2(control), gain_1/2(control), window_5/3(control), window_4/3(control), window_3/3(control), window_2/3(control), window_1/3(control)
  room_node/2(AIB) -> AIB/1, wall_3/4(AIB), wall_4/4(AIB), wall_5/4(AIB), wall_6/4(AIB), gain_2/1(AIB), gain_3/1(AIB), infiltration_2/1(AIB), infiltration_3/1(AIB), infiltration_4/1(AIB), infiltration_5/1(AIB), infiltration_1/1(AIB), gain_5/1(AIB), gain_4/1(AIB), gain_1/1(AIB), window_5/2(AIB), window_4/2(AIB), window_3/2(AIB), window_2/2(AIB), window_1/2(AIB), wall_2/4(AIB), wall_1/4(AIB)
  Mux/1 -> theta_out/1
  [theta_out_1] -> Mux/1
  [theta_out_2] -> Mux/2
  [theta_out_10] -> Mux/10
  [theta_out_9] -> Mux/9
  [theta_out_8] -> Mux/8
  [theta_out_7] -> Mux/7
  [theta_out_6] -> Mux/6
  [theta_out_5] -> Mux/5
  [theta_out_4] -> Mux/4
  [theta_out_3] -> Mux/3
  wall_2/2(theta_out) -> [theta_out_2]
  GDB/1 -> wall_1/2(GDB), wall_3/2(GDB), wall_4/2(GDB), wall_6/2(GDB), wall_5/2(GDB), wall_2/2(GDB)
  wall_3/2(theta_out) -> [theta_out_3]
  wall_4/2(theta_out) -> [theta_out_4]
  wall_5/2(theta_out) -> [theta_out_5]
  wall_6/2(theta_out) -> [theta_out_6]
  NDB/1 -> wall_1/3(NDB), wall_3/3(NDB), wall_4/3(NDB), wall_6/3(NDB), wall_5/3(NDB), wall_2/3(NDB)
  wall_1/1("[S]") -> Add1/1
  wall_6/1("[S]") -> Add1/6
  wall_2/1("[S]") -> Add1/2
  wall_3/1("[S]") -> Add1/3
  wall_4/1("[S]") -> Add1/4
  wall_5/1("[S]") -> Add1/5
  Add1/1 -> Add/2
  window_1/1("[S]") -> Add2/1
  window_5/1("[S]") -> Add2/5
  window_2/1("[S]") -> Add2/2
  window_3/1("[S]") -> Add2/3
  window_4/1("[S]") -> Add2/4
  Add2/1 -> Add/3
  gain_1/1("[S]") -> Add3/1
  gain_5/1("[S]") -> Add3/5
  gain_2/1("[S]") -> Add3/2
  gain_3/1("[S]") -> Add3/3
  gain_4/1("[S]") -> Add3/4
  Add3/1 -> Add/4
  infiltration_1/1("[S]") -> Add4/1
  infiltration_5/1("[S]") -> Add4/5
  infiltration_4/1("[S]") -> Add4/4
  infiltration_3/1("[S]") -> Add4/3
  infiltration_2/1("[S]") -> Add4/2
  Add4/1 -> Add/5

== system building_EXAMPLE_v1/BUILDING/ZONE_5 ==
  note: VECTOR theta_out
  note: NUMBEROFWALLSINZONES
  WDB : Inport
  GDB : Inport  Port=2
  NDB : Inport  Port=3
  S_in : Inport  Port=4
  Qdot_in : Inport  Port=5
  control : Inport  Port=6
  Add{,2..4} (4 alike) : Sum  Inputs=5
  Add1 : Sum  Inputs=6
  Mux : Mux  Inputs=10
  gain_1 : Subsystem  Variant=on  mask{zone=z.matrix_gains, gains=b.gains, subgain=1}
      mask init: same as building_EXAMPLE_v1/BUILDING/ZONE_1/gain_1
      mask Display:
      | fprintf('GAINS:\n')
      | fprintf('\n%s', ga.name)
  gain_2 : Subsystem  Variant=on  mask{zone=z.matrix_gains, gains=b.gains, subgain=2}
      mask init: same as building_EXAMPLE_v1/BUILDING/ZONE_1/gain_1
      mask Display:
      | fprintf('GAINS:\n')
      | fprintf('\n%s', ga.name)
  gain_3 : Subsystem  Variant=on  mask{zone=z.matrix_gains, gains=b.gains, subgain=3}
      mask init: same as building_EXAMPLE_v1/BUILDING/ZONE_1/gain_1
      mask Display:
      | fprintf('GAINS:\n')
      | fprintf('\n%s', ga.name)
  gain_4 : Subsystem  Variant=on  mask{zone=z.matrix_gains, gains=b.gains, subgain=4}
      mask init: same as building_EXAMPLE_v1/BUILDING/ZONE_1/gain_1
      mask Display:
      | fprintf('GAINS:\n')
      | fprintf('\n%s', ga.name)
  gain_5 : Subsystem  Variant=on  mask{zone=z.matrix_gains, gains=b.gains, subgain=4}
      mask init: same as building_EXAMPLE_v1/BUILDING/ZONE_1/gain_1
      mask Display:
      | fprintf('GAINS:\n')
      | fprintf('\n%s', ga.name)
  infiltration_1 : Subsystem  Variant=on  mask{zone=z.matrix_wi, window=1}
      mask init: same as building_EXAMPLE_v1/BUILDING/ZONE_1/infiltration_1
      mask Display:
      | fprintf('INFILTRATION:\n')
      | %fprintf('\n%s', const.name)
  infiltration_2 : Subsystem  Variant=on  mask{zone=z.matrix_wi, window=2}
      mask init: same as building_EXAMPLE_v1/BUILDING/ZONE_1/infiltration_1
      mask Display:
      | fprintf('INFILTRATION:\n')
      | %fprintf('\n%s', const.name)
  infiltration_3 : Subsystem  Variant=on  mask{zone=z.matrix_wi, window=3}
      mask init: same as building_EXAMPLE_v1/BUILDING/ZONE_1/infiltration_1
      mask Display:
      | fprintf('INFILTRATION:\n')
      | %fprintf('\n%s', const.name)
  infiltration_4 : Subsystem  Variant=on  mask{zone=z.matrix_wi, window=4}
      mask init: same as building_EXAMPLE_v1/BUILDING/ZONE_1/infiltration_1
      mask Display:
      | fprintf('INFILTRATION:\n')
      | %fprintf('\n%s', const.name)
  infiltration_5 : Subsystem  Variant=on  mask{zone=z.matrix_wi, window=5}
      mask init: same as building_EXAMPLE_v1/BUILDING/ZONE_1/infiltration_1
      mask Display:
      | fprintf('INFILTRATION:\n')
      | %fprintf('\n%s', const.name)
  room_node : Subsystem  Variant=on
  wall_1 : Subsystem  Variant=on  mask{zone=z.matrix_wd, construction=b.construction, wall=1}
      mask init: same as building_EXAMPLE_v1/BUILDING/ZONE_1/wall_1
      mask Display:
      | fprintf('CONSTRUCTION:\n')
      | fprintf('\n%s', const.name)
  wall_2 : Subsystem  Variant=on  mask{zone=z.matrix_wd, construction=b.construction, wall=2}
      mask init: same as building_EXAMPLE_v1/BUILDING/ZONE_1/wall_1
      mask Display:
      | fprintf('CONSTRUCTION:\n')
      | fprintf('\n%s', const.name)
  wall_3 : Subsystem  Variant=on  mask{zone=z.matrix_wd, construction=b.construction, wall=3}
      mask init: same as building_EXAMPLE_v1/BUILDING/ZONE_1/wall_1
      mask Display:
      | fprintf('CONSTRUCTION:\n')
      | fprintf('\n%s', const.name)
  wall_4 : Subsystem  Variant=on  mask{zone=z.matrix_wd, construction=b.construction, wall=4}
      mask init: same as building_EXAMPLE_v1/BUILDING/ZONE_1/wall_1
      mask Display:
      | fprintf('CONSTRUCTION:\n')
      | fprintf('\n%s', const.name)
  wall_5 : Subsystem  Variant=on  mask{zone=z.matrix_wd, construction=b.construction, wall=5}
      mask init: same as building_EXAMPLE_v1/BUILDING/ZONE_1/wall_1
      mask Display:
      | fprintf('CONSTRUCTION:\n')
      | fprintf('\n%s', const.name)
  wall_6 : Subsystem  Variant=on  mask{zone=z.matrix_wd, construction=b.construction, wall=6}
      mask init: same as building_EXAMPLE_v1/BUILDING/ZONE_1/wall_1
      mask Display:
      | fprintf('CONSTRUCTION:\n')
      | fprintf('\n%s', const.name)
  window_1 : Subsystem  Variant=on  mask{zone=z.matrix_wi, construction=b.construction, window=1}
      mask init: same as building_EXAMPLE_v1/BUILDING/ZONE_1/window_1
      mask Display:
      | fprintf('CONSTRUCTION:\n')
      | fprintf('\n%s', const.name)
  window_2 : Subsystem  Variant=on  mask{zone=z.matrix_wi, construction=b.construction, window=2}
      mask init: same as building_EXAMPLE_v1/BUILDING/ZONE_1/window_1
      mask Display:
      | fprintf('CONSTRUCTION:\n')
      | fprintf('\n%s', const.name)
  window_3 : Subsystem  Variant=on  mask{zone=z.matrix_wi, construction=b.construction, window=3}
      mask init: same as building_EXAMPLE_v1/BUILDING/ZONE_1/window_1
      mask Display:
      | fprintf('CONSTRUCTION:\n')
      | fprintf('\n%s', const.name)
  window_4 : Subsystem  Variant=on  mask{zone=z.matrix_wi, construction=b.construction, window=4}
      mask init: same as building_EXAMPLE_v1/BUILDING/ZONE_1/window_1
      mask Display:
      | fprintf('CONSTRUCTION:\n')
      | fprintf('\n%s', const.name)
  window_5 : Subsystem  Variant=on  mask{zone=z.matrix_wi, construction=b.construction, window=5}
      mask init: same as building_EXAMPLE_v1/BUILDING/ZONE_1/window_1
      mask Display:
      | fprintf('CONSTRUCTION:\n')
      | fprintf('\n%s', const.name)
  BDB : Outport
  AIB : Outport  Port=2
  theta_out : Outport  Port=3
  wires:
  WDB/1 -> wall_3/1(WDB), wall_4/1(WDB), wall_5/1(WDB), wall_6/1(WDB), window_1/1(WDB), window_4/1(WDB), infiltration_2/2(WDB), infiltration_3/2(WDB), infiltration_4/2(WDB), infiltration_5/2(WDB), infiltration_1/2(WDB), window_5/1(WDB), window_3/1(WDB), window_2/1(WDB), wall_2/1(WDB), wall_1/1(WDB)
  room_node/1(BDB) -> BDB/1
  S_in/1 -> Add/1
  Qdot_in/1 -> wall_1/5(Qdot_in), wall_3/5(Qdot_in), wall_4/5(Qdot_in), wall_6/5(Qdot_in), wall_5/5(Qdot_in), wall_2/5(Qdot_in)
  Add/1 -> room_node/1(sum([S]))
  room_node/3(Qdot_sol) -> wall_3/6(Qdot_sol), wall_4/6(Qdot_sol), wall_6/6(Qdot_sol), wall_5/6(Qdot_sol), wall_2/6(Qdot_sol), wall_1/6(Qdot_sol)
  wall_1/2(theta_out) -> [theta_out_1]
  control/1 -> gain_2/2(control), gain_3/2(control), infiltration_1/3(control), infiltration_2/3(control), infiltration_3/3(control), infiltration_4/3(control), infiltration_5/3(control), gain_5/2(control), gain_4/2(control), gain_1/2(control), window_5/3(control), window_4/3(control), window_3/3(control), window_2/3(control), window_1/3(control)
  room_node/2(AIB) -> AIB/1, wall_3/4(AIB), wall_4/4(AIB), wall_5/4(AIB), wall_6/4(AIB), gain_2/1(AIB), gain_3/1(AIB), infiltration_2/1(AIB), infiltration_3/1(AIB), infiltration_4/1(AIB), infiltration_5/1(AIB), infiltration_1/1(AIB), gain_5/1(AIB), gain_4/1(AIB), gain_1/1(AIB), window_5/2(AIB), window_4/2(AIB), window_3/2(AIB), window_2/2(AIB), window_1/2(AIB), wall_2/4(AIB), wall_1/4(AIB)
  Mux/1 -> theta_out/1
  [theta_out_1] -> Mux/1
  [theta_out_2] -> Mux/2
  [theta_out_10] -> Mux/10
  [theta_out_9] -> Mux/9
  [theta_out_8] -> Mux/8
  [theta_out_7] -> Mux/7
  [theta_out_6] -> Mux/6
  [theta_out_5] -> Mux/5
  [theta_out_4] -> Mux/4
  [theta_out_3] -> Mux/3
  wall_2/2(theta_out) -> [theta_out_2]
  GDB/1 -> wall_1/2(GDB), wall_3/2(GDB), wall_4/2(GDB), wall_6/2(GDB), wall_5/2(GDB), wall_2/2(GDB)
  wall_3/2(theta_out) -> [theta_out_3]
  wall_4/2(theta_out) -> [theta_out_4]
  wall_5/2(theta_out) -> [theta_out_5]
  wall_6/2(theta_out) -> [theta_out_6]
  NDB/1 -> wall_1/3(NDB), wall_3/3(NDB), wall_4/3(NDB), wall_6/3(NDB), wall_5/3(NDB), wall_2/3(NDB)
  wall_1/1("[S]") -> Add1/1
  wall_6/1("[S]") -> Add1/6
  wall_2/1("[S]") -> Add1/2
  wall_3/1("[S]") -> Add1/3
  wall_4/1("[S]") -> Add1/4
  wall_5/1("[S]") -> Add1/5
  Add1/1 -> Add/2
  window_1/1("[S]") -> Add2/1
  window_5/1("[S]") -> Add2/5
  window_2/1("[S]") -> Add2/2
  window_3/1("[S]") -> Add2/3
  window_4/1("[S]") -> Add2/4
  Add2/1 -> Add/3
  gain_1/1("[S]") -> Add3/1
  gain_5/1("[S]") -> Add3/5
  gain_2/1("[S]") -> Add3/2
  gain_3/1("[S]") -> Add3/3
  gain_4/1("[S]") -> Add3/4
  Add3/1 -> Add/4
  infiltration_1/1("[S]") -> Add4/1
  infiltration_5/1("[S]") -> Add4/5
  infiltration_4/1("[S]") -> Add4/4
  infiltration_3/1("[S]") -> Add4/3
  infiltration_2/1("[S]") -> Add4/2
  Add4/1 -> Add/5
